simulink model "SIM"  (R2020b)
settings: Solver=ode1  StartTime=0.0  StopTime=inf  FixedStep=0.005  RelTol=1e-3
values from neighbouring files (symbols this model uses):
  previous_input_to_hidden_layer = rand (K,1)* 0.2 - 0.1    [preparation.m]
  TableSIN = [0 0.0549778488291 0.109955562006 0.164933003878 0.219910038795 0.274886531105 0.32986234516 0.384837345313 0.439811395917 0.494784361331 0.549756105914 0.604726494028 ... (5001 elements, 5001x1)]    [TableSIN.mat]
  weights_Qj_model = rand (S,K)* 0.2 - 0.1    [preparation.m]
  weights_W2 = rand ( K+1 , R ) * 0.2 - 0.1    [preparation.m]
  weights_W3 = rand ( R+1 , W ) * 0.2 - 0.1    [preparation.m]
  weights_Wd_model = rand (K,1)* 0.2 - 0.1    [preparation.m]
  weights_Y1_model = rand (K,1)* 0.2 - 0.1    [preparation.m]
  weigths_W1 = rand ( S+1 , K ) * 0.2 - 0.1    [preparation.m]
undefined symbols (not defined in the file or in its folder): D, I, N, P, scaling_a, scaling_b, SkalB, SkalG, strengthening_PID, weights_W1_Model, weights_W2_Model, weights_Xj, WzmocnienieDoWyjscia
libraries: bur_blks x111, pid_lib x3
(part 2 of 2)

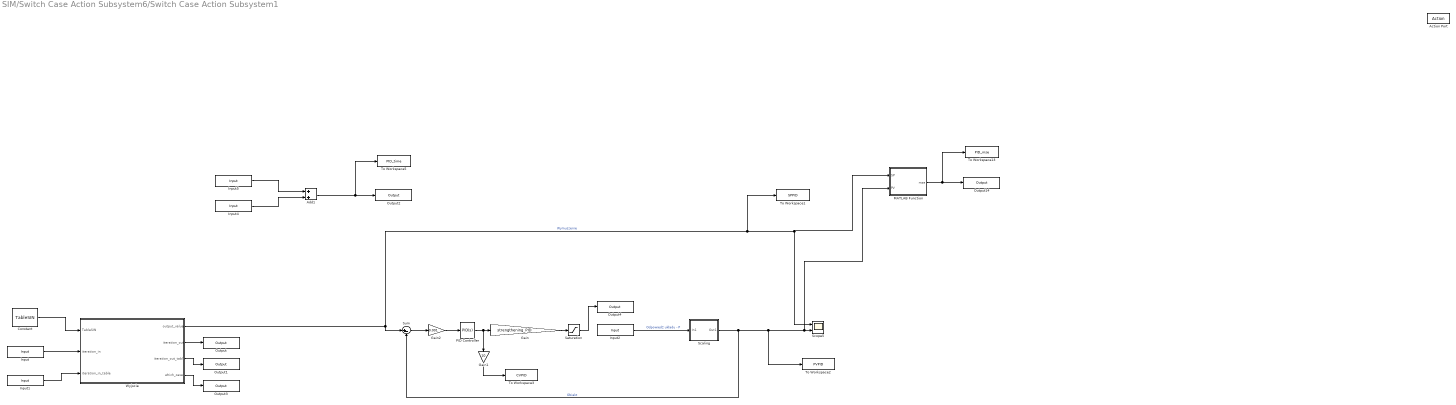
== system SIM/Switch Case Action Subsystem6/Switch Case Action Subsystem1 ==
  Action Port : ActionPort  ActionPortLabel=case [ 2 ]:
  Add1 : Sum
  Constant : Constant  Value=TableSIN
  Gain : Gain  Gain=strengthening_PID
  Gain1 : Gain  Gain=10
  Gain2 : Gain  Gain=0.001
  Input : bur_blks/Input  Tag=LOCAL REAL time_iterator  bur_var_name=time_iterator  bur_scope=LOCAL  bur_data_type=REAL  bur_init_value=-0.001  bur_init_value_bool=FALSE  bur_array_index=0  bur_var_memory=standard  bur_in_parameter=off  bur_AS_string=time_iterator : REAL := -0.001; (**)  bur_array_index_string=0
      settings: AttributesFormatString=%<Tag>  SourceProductName=B&R Automation Studio Toolbox
  Input1 : bur_blks/Input  Tag=LOCAL LREAL table_iterator  bur_var_name=table_iterator  bur_scope=LOCAL  bur_data_type=LREAL  bur_init_value=0  bur_init_value_bool=FALSE  bur_array_index=0  bur_var_memory=standard  bur_in_parameter=off  bur_AS_string=table_iterator : LREAL := 0; (**)  bur_array_index_string=0
      settings: AttributesFormatString=%<Tag>  SourceProductName=B&R Automation Studio Toolbox
  Input2 : bur_blks/Input  Tag=LOCAL LREAL a_input  bur_var_name=a_input  bur_scope=LOCAL  bur_data_type=LREAL  bur_init_value=0  bur_init_value_bool=FALSE  bur_array_index=0  bur_var_memory=standard  bur_in_parameter=off  bur_AS_string=a_input : LREAL := 0; (**)  bur_array_index_string=0
      settings: AttributesFormatString=%<Tag>  SourceProductName=B&R Automation Studio Toolbox
  Input4 : bur_blks/Input  Tag=LOCAL LREAL time  bur_var_name=time  bur_scope=LOCAL  bur_data_type=LREAL  bur_init_value=-0.001  bur_init_value_bool=FALSE  bur_array_index=0  bur_var_memory=standard  bur_in_parameter=off  bur_AS_string=time : LREAL := -0.001; (**)  bur_array_index_string=0
      settings: AttributesFormatString=%<Tag>  SourceProductName=B&R Automation Studio Toolbox
  Input5 : bur_blks/Input  Tag=LOCAL LREAL step  bur_var_name=step  bur_scope=LOCAL  bur_data_type=LREAL  bur_init_value=0  bur_init_value_bool=FALSE  bur_array_index=0  bur_var_memory=standard  bur_in_parameter=off  bur_AS_string=step : LREAL := 0; (**)  bur_array_index_string=0
      settings: AttributesFormatString=%<Tag>  SourceProductName=B&R Automation Studio Toolbox
  MATLAB Function : MATLAB Function  TreatAsAtomicUnit=on
  Output : bur_blks/Output  Tag=LOCAL REAL time_iterator  bur_var_name=time_iterator  bur_scope=LOCAL  bur_data_type=REAL  bur_init_value=0  bur_init_value_bool=FALSE  bur_array_index=0  bur_var_memory=standard  bur_AS_string=time_iterator : REAL := 0; (**)  bur_array_index_string=0
      settings: AttributesFormatString=%<Tag>  SourceProductName=B&R Automation Studio Toolbox
  Output1 : bur_blks/Output  Tag=LOCAL LREAL table_iterator  bur_var_name=table_iterator  bur_scope=LOCAL  bur_data_type=LREAL  bur_init_value=0  bur_init_value_bool=FALSE  bur_array_index=0  bur_var_memory=standard  bur_AS_string=table_iterator : LREAL := 0; (**)  bur_array_index_string=0
      settings: AttributesFormatString=%<Tag>  SourceProductName=B&R Automation Studio Toolbox
  Output14 : bur_blks/Output  Tag=LOCAL LREAL PID_mse  bur_var_name=PID_mse  bur_scope=LOCAL  bur_data_type=LREAL  bur_init_value=0  bur_init_value_bool=FALSE  bur_array_index=0  bur_var_memory=standard  bur_AS_string=PID_mse : LREAL := 0; (**)  bur_array_index_string=0
      settings: AttributesFormatString=%<Tag>  SourceProductName=B&R Automation Studio Toolbox
  Output2 : bur_blks/Output  Tag=LOCAL LREAL time  bur_var_name=time  bur_scope=LOCAL  bur_data_type=LREAL  bur_init_value=0  bur_init_value_bool=FALSE  bur_array_index=0  bur_var_memory=standard  bur_AS_string=time : LREAL := 0; (**)  bur_array_index_string=0
      settings: AttributesFormatString=%<Tag>  SourceProductName=B&R Automation Studio Toolbox
  Output3 : bur_blks/Output  Tag=LOCAL LREAL Case2  bur_var_name=Case2  bur_scope=LOCAL  bur_data_type=LREAL  bur_init_value=0  bur_init_value_bool=FALSE  bur_array_index=0  bur_var_memory=standard  bur_array_index_string=0
      settings: AttributesFormatString=%<Tag>  SourceProductName=B&R Automation Studio Toolbox
  Output4 : bur_blks/Output  Tag=LOCAL LREAL a_output  bur_var_name=a_output  bur_scope=LOCAL  bur_data_type=LREAL  bur_init_value=0  bur_init_value_bool=FALSE  bur_array_index=0  bur_var_memory=standard  bur_AS_string=a_output : LREAL := 0; (**)  bur_array_index_string=0
      settings: AttributesFormatString=%<Tag>  SourceProductName=B&R Automation Studio Toolbox
  PID Controller : pid_lib/PID Controller  Controller=PID  Form=Parallel  TimeDomain=Continuous-time  UseExternalTs=off  SampleTime=-1  IntegratorMethod=Forward Euler  FilterMethod=Forward Euler  ControllerParametersSource=internal  P=P  I=I  D=D  UseFilter=on  N=N  TunerSelectOption=Transfer Function Based (PID Tuner App)  InitialConditionSource=internal  InitialConditionForIntegrator=0  InitialConditionForFilter=0  DifferentiatorICPrevScaledInput=0  ExternalReset=none  TrackingMode=off  Kt=1  LimitOutput=on  SatLimitsSource=internal  UpperSaturationLimit=1  LowerSaturationLimit=-1  LinearizeAsGain=on  AntiWindupMode=clamping  Kb=1  POutMin=[]  POutMax=[]  IOutMin=[]  IOutMax=[]  DOutMin=[]  DOutMax=[]  NOutMin=[]  NOutMax=[]  SumOutMin=[]  SumOutMax=[]  SaturationOutMin=[]  SaturationOutMax=[]  PParamMin=[]  PParamMax=[]  IParamMin=[]  IParamMax=[]  DParamMin=[]  DParamMax=[]  NParamMin=[]  NParamMax=[]  KbParamMin=[]  KbParamMax=[]  KtParamMin=[]  KtParamMax=[]  KbOutMin=[]  KbOutMax=[]  KtOutMin=[]  KtOutMax=[]  IntegratorOutMin=[]  IntegratorOutMax=[]  FilterOutMin=[]  FilterOutMax=[]  SumI1OutMin=[]  SumI1OutMax=[]  SumI2OutMin=[]  SumI2OutMax=[]  SumI3OutMin=[]  SumI3OutMax=[]  SumI4OutMin=[]  SumI4OutMax=[]  SumDOutMin=[]  SumDOutMax=[]  DifferentiatorOutMin=[]  DifferentiatorOutMax=[]  FilterDiffOutCoefMin=[]  FilterDiffOutCoefMax=[]  ReciprocalOutMin=[]  ReciprocalOutMax=[]  SumDenOutMin=[]  SumDenOutMax=[]  SumNumOutMin=[]  SumNumOutMax=[]  DivideOutMin=[]  DivideOutMax=[]  UdiffTsProdOutMin=[]  UdiffTsProdOutMax=[]  NTsProdOutMin=[]  NTsProdOutMax=[]  UintegralTsProdOutMin=[]  UintegralTsProdOutMax=[]  UngainTsProdOutMin=[]  UngainTsProdOutMax=[]  IntegratorContinuousStateAttributes=''  IntegratorStateMustResolveToSignalObject=off  IntegratorRTWStateStorageClass=Auto  FilterContinuousStateAttributes=''  FilterStateMustResolveToSignalObject=off  FilterRTWStateStorageClass=Auto  ParallelPVariant=InternalParameters  IdealPVariant=Disabled  IVariant=InternalParameters  DVariant=InternalParameters  IntegratorVariant=Continuous  SatVariant=Enabled  AWVariant=ContClampingParallel  PCopyVariant=Disabled  TRVariant=Disabled  FdbkBlocksVariant=Forward  IdealPFdbkVariant=Disabled  SatFdbkVariant=Disabled  DerivativeFilterVariant=ContFilter  NVariant=InternalParameters  NCopyVariant=Disabled  FilterICVariant=InternalICsFilter  IntegratorICVariant=InternalICs  ExternalResetVariant=Disabled  TRSumVariant=Passthrough  SumFdbkVariant=Disabled  SumVariant=Sum_PID  TsampFilterVariant=InternalTs  TsampNgainVariant=Passthrough  TsampIntegralVariant=Passthrough  ExternalSaturationOutDataTypeStr=Inherit: Same as second input
  Saturation : Saturate  UpperLimit=32767  LowerLimit=-32767
  Scaling : Subsystem
  Scope5 : Scope  NumInputPorts=2
  Sum : Sum  Inputs=|+-
  To Workspace1 : ToWorkspace  VariableName=SPPID  SampleTime=-1
  To Workspace13 : ToWorkspace  VariableName=PID_mse  SampleTime=-1
  To Workspace2 : ToWorkspace  VariableName=PVPID  SampleTime=-1
  To Workspace3 : ToWorkspace  VariableName=CVPID  SampleTime=-1
  To Workspace5 : ToWorkspace  VariableName=PID_time  SampleTime=-1
  Wyjscie : MATLAB Function  TreatAsAtomicUnit=on
  wires:
  Input4/1 -> Add1/2
  Add1/1 -> To Workspace5/1, Output2/1
  Input5/1 -> Add1/1
  Sum/1 -> Gain2/1
  Wyjscie/1(output_value) -> Sum/1, To Workspace1/1, Scope5/1, MATLAB Function/1(SP)  "Wymuszenie"
  PID Controller/1 -> Gain1/1, Gain/1
  Input/1 -> Wyjscie/2(iteration_in)
  Wyjscie/4(which_case) -> Output3/1
  Wyjscie/3(iteration_out_table) -> Output1/1
  Wyjscie/2(iteration_out) -> Output/1
  Constant/1 -> Wyjscie/1(TableSIN)
  Scaling/1(Out1) -> Sum/2, To Workspace2/1, MATLAB Function/2(PV), Scope5/2  "Obiekt"
  MATLAB Function/1(mse) -> To Workspace13/1, Output14/1
  Input2/1 -> Scaling/1(In1)  "Odpowiedź układu - P"
  Gain/1 -> Saturation/1
  Saturation/1 -> Output4/1
  Gain2/1 -> PID Controller/1
  Gain1/1 -> To Workspace3/1
  Input1/1 -> Wyjscie/3(iteration_in_table)

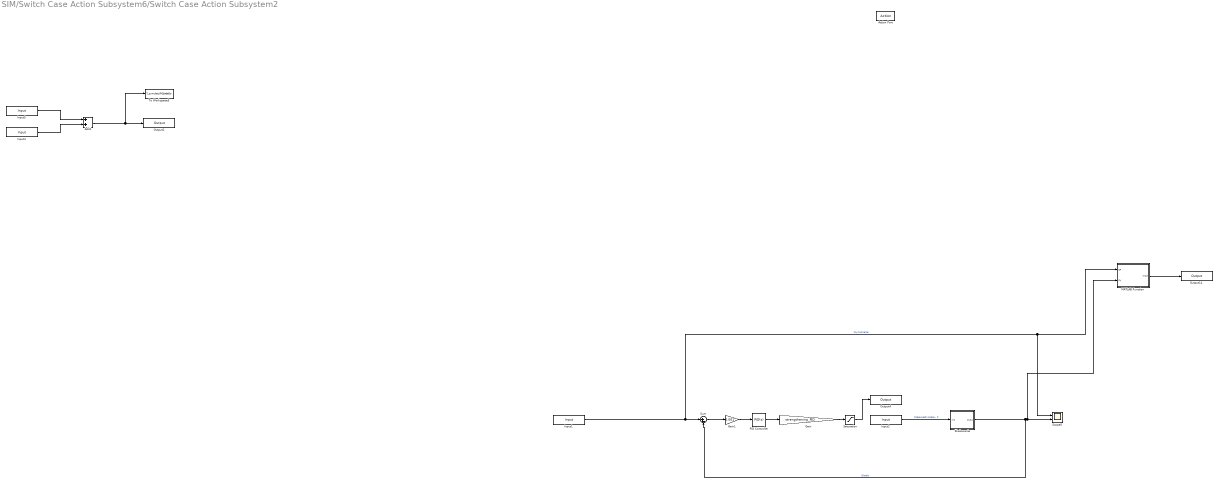
== system SIM/Switch Case Action Subsystem6/Switch Case Action Subsystem2 ==
  Action Port : ActionPort  ActionPortLabel=case [ 3 ]:
  Add1 : Sum
  Gain : Gain  Gain=strengthening_PID
  Gain1 : Gain  Gain=0.001
  Input1 : bur_blks/Input  Tag=LOCAL LREAL PID_reference  bur_var_name=PID_reference  bur_scope=LOCAL  bur_data_type=LREAL  bur_init_value=0  bur_init_value_bool=FALSE  bur_array_index=0  bur_var_memory=standard  bur_in_parameter=off  bur_AS_string=PID_reference : LREAL := 0; (**)  bur_array_index_string=0
      settings: AttributesFormatString=%<Tag>  SourceProductName=B&R Automation Studio Toolbox
  Input2 : bur_blks/Input  Tag=LOCAL LREAL a_input  bur_var_name=a_input  bur_scope=LOCAL  bur_data_type=LREAL  bur_init_value=0  bur_init_value_bool=FALSE  bur_array_index=0  bur_var_memory=standard  bur_in_parameter=off  bur_AS_string=a_input : LREAL := 0; (**)  bur_array_index_string=0
      settings: AttributesFormatString=%<Tag>  SourceProductName=B&R Automation Studio Toolbox
  Input4 : bur_blks/Input  Tag=LOCAL LREAL time  bur_var_name=time  bur_scope=LOCAL  bur_data_type=LREAL  bur_init_value=-0.001  bur_init_value_bool=FALSE  bur_array_index=0  bur_var_memory=standard  bur_in_parameter=off  bur_AS_string=time : LREAL := -0.001; (**)  bur_array_index_string=0
      settings: AttributesFormatString=%<Tag>  SourceProductName=B&R Automation Studio Toolbox
  Input5 : bur_blks/Input  Tag=LOCAL LREAL step  bur_var_name=step  bur_scope=LOCAL  bur_data_type=LREAL  bur_init_value=0  bur_init_value_bool=FALSE  bur_array_index=0  bur_var_memory=standard  bur_in_parameter=off  bur_AS_string=step : LREAL := 0; (**)  bur_array_index_string=0
      settings: AttributesFormatString=%<Tag>  SourceProductName=B&R Automation Studio Toolbox
  MATLAB Function : MATLAB Function  TreatAsAtomicUnit=on
  Output14 : bur_blks/Output  Tag=LOCAL LREAL PID_mse  bur_var_name=PID_mse  bur_scope=LOCAL  bur_data_type=LREAL  bur_init_value=0  bur_init_value_bool=FALSE  bur_array_index=0  bur_var_memory=standard  bur_AS_string=PID_mse : LREAL := 0; (**)  bur_array_index_string=0
      settings: AttributesFormatString=%<Tag>  SourceProductName=B&R Automation Studio Toolbox
  Output2 : bur_blks/Output  Tag=LOCAL LREAL time  bur_var_name=time  bur_scope=LOCAL  bur_data_type=LREAL  bur_init_value=0  bur_init_value_bool=FALSE  bur_array_index=0  bur_var_memory=standard  bur_AS_string=time : LREAL := 0; (**)  bur_array_index_string=0
      settings: AttributesFormatString=%<Tag>  SourceProductName=B&R Automation Studio Toolbox
  Output4 : bur_blks/Output  Tag=LOCAL LREAL a_output  bur_var_name=a_output  bur_scope=LOCAL  bur_data_type=LREAL  bur_init_value=0  bur_init_value_bool=FALSE  bur_array_index=0  bur_var_memory=standard  bur_AS_string=a_output : LREAL := 0; (**)  bur_array_index_string=0
      settings: AttributesFormatString=%<Tag>  SourceProductName=B&R Automation Studio Toolbox
  PID Controller : pid_lib/PID Controller  Controller=PID  Form=Parallel  TimeDomain=Continuous-time  UseExternalTs=off  SampleTime=-1  IntegratorMethod=Forward Euler  FilterMethod=Forward Euler  ControllerParametersSource=internal  P=P  I=I  D=D  UseFilter=on  N=N  TunerSelectOption=Transfer Function Based (PID Tuner App)  InitialConditionSource=internal  InitialConditionForIntegrator=0  InitialConditionForFilter=0  DifferentiatorICPrevScaledInput=0  ExternalReset=none  TrackingMode=off  Kt=1  LimitOutput=on  SatLimitsSource=internal  UpperSaturationLimit=1  LowerSaturationLimit=-1  LinearizeAsGain=on  AntiWindupMode=clamping  Kb=1  POutMin=[]  POutMax=[]  IOutMin=[]  IOutMax=[]  DOutMin=[]  DOutMax=[]  NOutMin=[]  NOutMax=[]  SumOutMin=[]  SumOutMax=[]  SaturationOutMin=[]  SaturationOutMax=[]  PParamMin=[]  PParamMax=[]  IParamMin=[]  IParamMax=[]  DParamMin=[]  DParamMax=[]  NParamMin=[]  NParamMax=[]  KbParamMin=[]  KbParamMax=[]  KtParamMin=[]  KtParamMax=[]  KbOutMin=[]  KbOutMax=[]  KtOutMin=[]  KtOutMax=[]  IntegratorOutMin=[]  IntegratorOutMax=[]  FilterOutMin=[]  FilterOutMax=[]  SumI1OutMin=[]  SumI1OutMax=[]  SumI2OutMin=[]  SumI2OutMax=[]  SumI3OutMin=[]  SumI3OutMax=[]  SumI4OutMin=[]  SumI4OutMax=[]  SumDOutMin=[]  SumDOutMax=[]  DifferentiatorOutMin=[]  DifferentiatorOutMax=[]  FilterDiffOutCoefMin=[]  FilterDiffOutCoefMax=[]  ReciprocalOutMin=[]  ReciprocalOutMax=[]  SumDenOutMin=[]  SumDenOutMax=[]  SumNumOutMin=[]  SumNumOutMax=[]  DivideOutMin=[]  DivideOutMax=[]  UdiffTsProdOutMin=[]  UdiffTsProdOutMax=[]  NTsProdOutMin=[]  NTsProdOutMax=[]  UintegralTsProdOutMin=[]  UintegralTsProdOutMax=[]  UngainTsProdOutMin=[]  UngainTsProdOutMax=[]  IntegratorContinuousStateAttributes=''  IntegratorStateMustResolveToSignalObject=off  IntegratorRTWStateStorageClass=Auto  FilterContinuousStateAttributes=''  FilterStateMustResolveToSignalObject=off  FilterRTWStateStorageClass=Auto  ParallelPVariant=InternalParameters  IdealPVariant=Disabled  IVariant=InternalParameters  DVariant=InternalParameters  IntegratorVariant=Continuous  SatVariant=Enabled  AWVariant=ContClampingParallel  PCopyVariant=Disabled  TRVariant=Disabled  FdbkBlocksVariant=Forward  IdealPFdbkVariant=Disabled  SatFdbkVariant=Disabled  DerivativeFilterVariant=ContFilter  NVariant=InternalParameters  NCopyVariant=Disabled  FilterICVariant=InternalICsFilter  IntegratorICVariant=InternalICs  ExternalResetVariant=Disabled  TRSumVariant=Passthrough  SumFdbkVariant=Disabled  SumVariant=Sum_PID  TsampFilterVariant=InternalTs  TsampNgainVariant=Passthrough  TsampIntegralVariant=Passthrough  ExternalSaturationOutDataTypeStr=Inherit: Same as second input
  Saturation : Saturate  UpperLimit=32767  LowerLimit=-32767
  Scope5 : Scope  NumInputPorts=2
  Skalowanie : Subsystem
  Sum : Sum  Inputs=|+-
  To Workspace5 : ToWorkspace  VariableName=T_symulacjiPIDJadeDo  SampleTime=-1
  wires:
  Input5/1 -> Add1/1
  Add1/1 -> To Workspace5/1, Output2/1
  Input4/1 -> Add1/2
  Sum/1 -> Gain1/1
  MATLAB Function/1(mse) -> Output14/1
  Input1/1 -> MATLAB Function/1(SP), Scope5/1, Sum/1  "Wymuszenie"
  Skalowanie/1(Out1) -> Sum/2, MATLAB Function/2(PV), Scope5/2  "Obiekt"
  Saturation/1 -> Output4/1
  PID Controller/1 -> Gain/1
  Gain/1 -> Saturation/1
  Input2/1 -> Skalowanie/1(In1)  "Odpowiedź układu - P"
  Gain1/1 -> PID Controller/1

== system SIM/Switch Case Action Subsystem6/Switch Case Action Subsystem3 ==
  Action Port : ActionPort  ActionPortLabel=default:
  Constant3 : Constant  Value=-1
  Constant5 : Constant  Value=0
  Constant8 : Constant  Value=-0.001
  Output10 : bur_blks/Output  Tag=LOCAL LREAL time_iterator  bur_var_name=time_iterator  bur_scope=LOCAL  bur_data_type=LREAL  bur_init_value=0  bur_init_value_bool=FALSE  bur_array_index=0  bur_var_memory=standard  bur_AS_string=time_iterator : LREAL := 0; (**)  bur_array_index_string=0
      settings: AttributesFormatString=%<Tag>  SourceProductName=B&R Automation Studio Toolbox
  Output13 : bur_blks/Output  Tag=LOCAL LREAL time  bur_var_name=time  bur_scope=LOCAL  bur_data_type=LREAL  bur_init_value=0  bur_init_value_bool=FALSE  bur_array_index=0  bur_var_memory=standard  bur_AS_string=time : LREAL := 0; (**)  bur_array_index_string=0
      settings: AttributesFormatString=%<Tag>  SourceProductName=B&R Automation Studio Toolbox
  Output9 : bur_blks/Output  Tag=LOCAL LREAL table_sq_iterator  bur_var_name=table_sq_iterator  bur_scope=LOCAL  bur_data_type=LREAL  bur_init_value=0  bur_init_value_bool=FALSE  bur_array_index=0  bur_var_memory=standard  bur_AS_string=table_sq_iterator : LREAL := 0; (**)  bur_array_index_string=0
      settings: AttributesFormatString=%<Tag>  SourceProductName=B&R Automation Studio Toolbox
  wires:
  Constant3/1 -> Output10/1
  Constant5/1 -> Output9/1
  Constant8/1 -> Output13/1

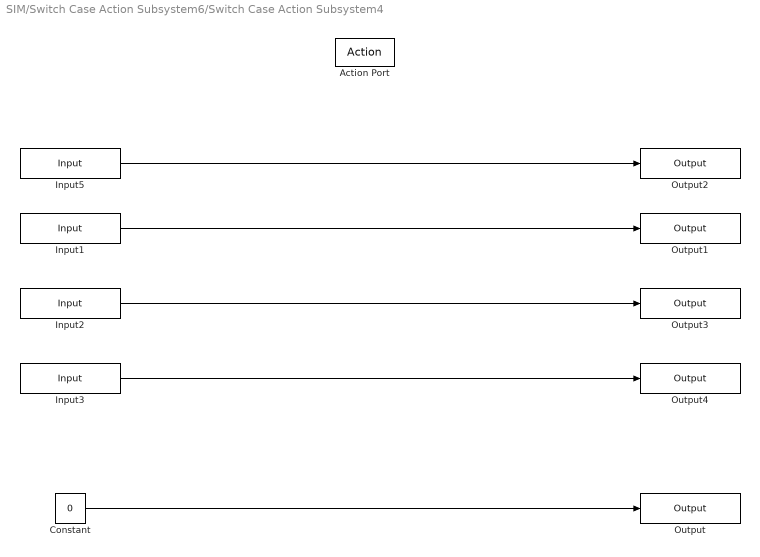
== system SIM/Switch Case Action Subsystem6/Switch Case Action Subsystem4 ==
  Action Port : ActionPort  ActionPortLabel=case [ 1 ]:
  Constant : Constant  Value=0
  Input1 : bur_blks/Input  Tag=LOCAL LREAL new_I  bur_var_name=new_I  bur_scope=LOCAL  bur_data_type=LREAL  bur_init_value=31.35  bur_init_value_bool=FALSE  bur_array_index=0  bur_var_memory=standard  bur_in_parameter=off  bur_AS_string=new_I : LREAL := 31.35; (**)  bur_array_index_string=0
      settings: AttributesFormatString=%<Tag>  SourceProductName=B&R Automation Studio Toolbox
  Input2 : bur_blks/Input  Tag=LOCAL LREAL new_D  bur_var_name=new_D  bur_scope=LOCAL  bur_data_type=LREAL  bur_init_value=0.0076  bur_init_value_bool=FALSE  bur_array_index=0  bur_var_memory=standard  bur_in_parameter=off  bur_AS_string=new_D : LREAL := 0.0076; (**)  bur_array_index_string=0
      settings: AttributesFormatString=%<Tag>  SourceProductName=B&R Automation Studio Toolbox
  Input3 : bur_blks/Input  Tag=LOCAL LREAL new_N  bur_var_name=new_N  bur_scope=LOCAL  bur_data_type=LREAL  bur_init_value=1  bur_init_value_bool=FALSE  bur_array_index=0  bur_var_memory=standard  bur_in_parameter=off  bur_AS_string=new_N : LREAL := 1; (**)  bur_array_index_string=0
      settings: AttributesFormatString=%<Tag>  SourceProductName=B&R Automation Studio Toolbox
  Input5 : bur_blks/Input  Tag=LOCAL LREAL new_P  bur_var_name=new_P  bur_scope=LOCAL  bur_data_type=LREAL  bur_init_value=130  bur_init_value_bool=FALSE  bur_array_index=0  bur_var_memory=standard  bur_in_parameter=off  bur_AS_string=new_P : LREAL := 130; (**)  bur_array_index_string=0
      settings: AttributesFormatString=%<Tag>  SourceProductName=B&R Automation Studio Toolbox
  Output : bur_blks/Output  Tag=LOCAL LREAL Case2  bur_var_name=Case2  bur_scope=LOCAL  bur_data_type=LREAL  bur_init_value=0  bur_init_value_bool=FALSE  bur_array_index=0  bur_var_memory=standard  bur_array_index_string=0
      settings: AttributesFormatString=%<Tag>  SourceProductName=B&R Automation Studio Toolbox
  Output1 : bur_blks/Output  Tag=LOCAL LREAL I  bur_var_name=I  bur_scope=LOCAL  bur_data_type=LREAL  bur_init_value=0  bur_init_value_bool=FALSE  bur_array_index=0  bur_var_memory=standard  bur_array_index_string=0
      settings: AttributesFormatString=%<Tag>  SourceProductName=B&R Automation Studio Toolbox
  Output2 : bur_blks/Output  Tag=LOCAL LREAL P  bur_var_name=P  bur_scope=LOCAL  bur_data_type=LREAL  bur_init_value=0  bur_init_value_bool=FALSE  bur_array_index=0  bur_var_memory=standard  bur_array_index_string=0
      settings: AttributesFormatString=%<Tag>  SourceProductName=B&R Automation Studio Toolbox
  Output3 : bur_blks/Output  Tag=LOCAL LREAL D  bur_var_name=D  bur_scope=LOCAL  bur_data_type=LREAL  bur_init_value=0  bur_init_value_bool=FALSE  bur_array_index=0  bur_var_memory=standard  bur_array_index_string=0
      settings: AttributesFormatString=%<Tag>  SourceProductName=B&R Automation Studio Toolbox
  Output4 : bur_blks/Output  Tag=LOCAL LREAL N  bur_var_name=N  bur_scope=LOCAL  bur_data_type=LREAL  bur_init_value=0  bur_init_value_bool=FALSE  bur_array_index=0  bur_var_memory=standard  bur_array_index_string=0
      settings: AttributesFormatString=%<Tag>  SourceProductName=B&R Automation Studio Toolbox
  wires:
  Constant/1 -> Output/1
  Input5/1 -> Output2/1
  Input1/1 -> Output1/1
  Input2/1 -> Output3/1
  Input3/1 -> Output4/1

== system SIM/Switch Case Action Subsystem4/Switch Case Action Subsystem1/Denormalisation ==
  u : Inport
  Gain1 : Gain  Gain=-1
  Input : bur_blks/Input  Tag=LOCAL LREAL normalisation  bur_var_name=normalisation  bur_scope=LOCAL  bur_data_type=LREAL  bur_init_value=0  bur_init_value_bool=FALSE  bur_array_index=0  bur_var_memory=standard  bur_in_parameter=off  bur_AS_string=normalisation : LREAL := 0; (**)  bur_array_index_string=0
      settings: AttributesFormatString=%<Tag>  SourceProductName=B&R Automation Studio Toolbox
  Input1 : bur_blks/Input  Tag=LOCAL LREAL normalisation  bur_var_name=normalisation  bur_scope=LOCAL  bur_data_type=LREAL  bur_init_value=0  bur_init_value_bool=FALSE  bur_array_index=0  bur_var_memory=standard  bur_in_parameter=off  bur_AS_string=normalisation : LREAL := 0; (**)  bur_array_index_string=0
      settings: AttributesFormatString=%<Tag>  SourceProductName=B&R Automation Studio Toolbox
  MATLAB Function : MATLAB Function  TreatAsAtomicUnit=on
  Xods : Outport
  wires:
  Input1/1 -> Gain1/1
  u/1 -> MATLAB Function/1(Xprze)
  MATLAB Function/1(Xods) -> Xods/1
  Input/1 -> MATLAB Function/2(Xmax)
  Gain1/1 -> MATLAB Function/3(Xmin)

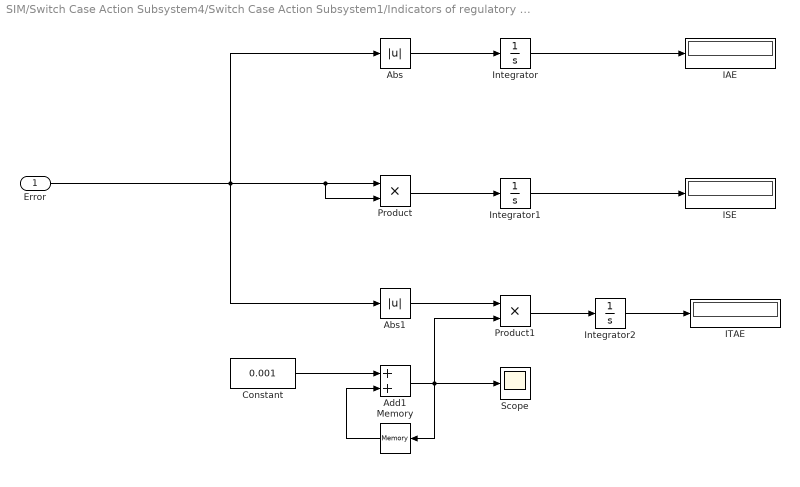
== system SIM/Switch Case Action Subsystem4/Switch Case Action Subsystem1/Indicators of regulatory quality ==
  Error : Inport
  Abs : Abs
  Abs1 : Abs
  Add1 : Sum
  Constant : Constant  Value=0.001
  IAE : Display
  ISE : Display
  ITAE : Display
  Integrator : Integrator
  Integrator1 : Integrator
  Integrator2 : Integrator
  Memory : Memory
  Product : Product
  Product1 : Product
  Scope : Scope
  wires:
  Error/1 -> Abs1/1, Product/2, Product/1, Abs/1
  Abs/1 -> Integrator/1
  Integrator/1 -> IAE/1
  Product/1 -> Integrator1/1
  Integrator1/1 -> ISE/1
  Abs1/1 -> Product1/1
  Constant/1 -> Add1/1
  Add1/1 -> Scope/1, Product1/2, Memory/1
  Product1/1 -> Integrator2/1
  Memory/1 -> Add1/2
  Integrator2/1 -> ITAE/1

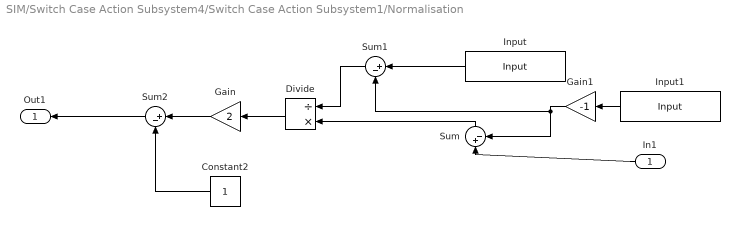
== system SIM/Switch Case Action Subsystem4/Switch Case Action Subsystem1/Normalisation ==
  In1 : Inport
  Constant2 : Constant
  Divide : Product  Inputs=/*
  Gain : Gain  Gain=2
  Gain1 : Gain  Gain=-1
  Input : bur_blks/Input  Tag=LOCAL LREAL normalisation  bur_var_name=normalisation  bur_scope=LOCAL  bur_data_type=LREAL  bur_init_value=0  bur_init_value_bool=FALSE  bur_array_index=0  bur_var_memory=standard  bur_in_parameter=off  bur_AS_string=normalisation : LREAL := 0; (**)  bur_array_index_string=0
      settings: AttributesFormatString=%<Tag>  SourceProductName=B&R Automation Studio Toolbox
  Input1 : bur_blks/Input  Tag=LOCAL LREAL normalisation  bur_var_name=normalisation  bur_scope=LOCAL  bur_data_type=LREAL  bur_init_value=0  bur_init_value_bool=FALSE  bur_array_index=0  bur_var_memory=standard  bur_in_parameter=off  bur_AS_string=normalisation : LREAL := 0; (**)  bur_array_index_string=0
      settings: AttributesFormatString=%<Tag>  SourceProductName=B&R Automation Studio Toolbox
  Sum : Sum  Inputs=|+-
  Sum1 : Sum  Inputs=|+-
  Sum2 : Sum  Inputs=|+-
  Out1 : Outport
  wires:
  In1/1 -> Sum/1
  Divide/1 -> Gain/1
  Sum/1 -> Divide/2
  Sum1/1 -> Divide/1
  Gain/1 -> Sum2/1
  Sum2/1 -> Out1/1
  Constant2/1 -> Sum2/2
  Input/1 -> Sum1/1
  Input1/1 -> Gain1/1
  Gain1/1 -> Sum/2, Sum1/2

== system SIM/Switch Case Action Subsystem4/Switch Case Action Subsystem1/Skalowanie3 ==
  In1 : Inport
  Add : Sum
  Constant : Constant  Value=SkalB
  Gain : Gain  Gain=SkalG
  Out1 : Outport
  wires:
  In1/1 -> Gain/1
  Gain/1 -> Add/2
  Add/1 -> Out1/1
  Constant/1 -> Add/1

== system SIM/Switch Case Action Subsystem6/Switch Case Action Subsystem1/Scaling ==
  In1 : Inport
  Add : Sum
  Constant : Constant  Value=scaling_b
  Gain : Gain  Gain=scaling_a
  Out1 : Outport
  wires:
  In1/1 -> Gain/1
  Gain/1 -> Add/2
  Add/1 -> Out1/1
  Constant/1 -> Add/1

== system SIM/Switch Case Action Subsystem6/Switch Case Action Subsystem2/Skalowanie ==
  In1 : Inport
  Add : Sum
  Constant : Constant  Value=scaling_b
  Gain : Gain  Gain=scaling_a
  Out1 : Outport
  wires:
  In1/1 -> Gain/1
  Gain/1 -> Add/2
  Add/1 -> Out1/1
  Constant/1 -> Add/1

== matlab function SIM/Switch Case Action Subsystem/MATLAB Function ==
  data: u input; max_output output; max_actual_output input; min_actual_output input; min_output output
function [max_output,min_output] = fcn(u,max_actual_output,min_actual_output)

max_output = max_actual_output;
min_output = min_actual_output;

if max_actual_output < u
   
    max_output = u;
    
end

if min_actual_output > u
   
    min_output = u;

end

    
end

== matlab function SIM/Switch Case Action Subsystem3/MATLAB Function ==
  data: scaling_a output; max_output input; min_output input; scaling_b output; which_case output
function [scaling_a,scaling_b,which_case] = fcn(max_output,min_output)

MAX = 67.75;
MIN = -67.75;

scaling_a = (MAX-MIN)/(max_output - min_output);
scaling_b = MAX - scaling_a*max_output;

which_case = 0;

end

== matlab function SIM/Switch Case Action Subsystem2/MATLAB Function1 ==
  data: T_symulacji input; Czy_koniec output
function Czy_koniec = fcn(T_symulacji)

Czy_koniec = 0;

if T_symulacji > 3
    
    Czy_koniec = 1;
end

== matlab function SIM/Switch Case Action Subsystem4/Switch Case Action Subsystem1/DRNN ==
  data: E input; reference_signal input; y output; weights_W1 input; weights_W2 input; weights_Wd_model input; weights_Xj_model input; previous_input_to_hidden_layer input; weights_Qj_model input; weights_W1_after output; weights_W2_after output; weights_Wd_after output; MSEOUT output; Xj_after output; Pj_after output; Qj_after output; previous_output_of_object_d1 input; previous_output_of_object_d2 input; iteration_before input; iteration_after output; output_of_hidden_layer output
function [y,weights_W1_after,weights_W2_after, weights_Wd_after,MSEOUT,Xj_after,Pj_after,Qj_after,iteration_after,output_of_hidden_layer] = ...
    fcn(E,reference_signal,weights_W1,weights_W2,weights_Wd_model,weights_Xj_model,previous_input_to_hidden_layer,weights_Qj_model,...
    previous_output_of_object_d1,previous_output_of_object_d2,iteration_before)

function [ W1po, W2po, Wdpo, MSE ] = ucz2 ( weights_W1_before , weights_W2_before , weights_Wd_before , input_to_network, previous_input_to_hidden_layer, Qjd , Xjd)
W1 = weights_W1_before ;
W2 = weights_W2_before ;
Wd = weights_Wd_before;
Xj = Xjd;

X = input_to_network; % wejścia sieci
[ Y1 , Y2, Xjpo] = dzialaj2 ( W1 , W2 , Wd , X , Xj) ;
X1 = [ X ] ; % wejścia warstwy 1
X2 = [ Y1 ] ; % wejścia warstwy 2
D2 = E; % oblicz błędy dla warstwy 2
E2 = D2; % błąd„wewnętrzny” warstwy 2
MSE = 0.5*D2'*D2;

coefficient = 1.5;
countofneurons = 15;

DerivativeUcAfterW2 = X2;
dW2 = DerivativeUcAfterW2;
W2 = W2 + (coefficient/(countofneurons))*dW2*E2';
wspUcz2warstwy = coefficient/(countofneurons);

W2max = max(abs(W2));
Imax = max(abs(X));

DerivativeUcAfterWd = (1 - Y1.*Y1);
%dWd = DerivativeUcAfterWd.*(Xjd + Wd.*Pjd);
dWd = (Xjd + previous_input_to_hidden_layer.*Wd).*(DerivativeUcAfterWd.*W2);
Pj_after = dWd;
Wd = Wd + (coefficient/(countofneurons*W2max*W2max))*dWd*E2;
wspUczPetli = coefficient/(countofneurons*W2max*W2max);
Wd(Wd>1)=1;
Wd(Wd<-1)=-1;

DerivativeUcAfterW1 = (1 - Y1.*Y1);
dW1 = (X1 + Qjd*Wd)*(DerivativeUcAfterW1.*W2)';
Qj_after = dW1;
W1 = W1 + (coefficient/(countofneurons*W2max*W2max*Imax*Imax))*dW1*E2;
wspUcz1warstwy = coefficient/(countofneurons*W2max*W2max*Imax*Imax);

W1po = W1 ;
W2po = W2 ;
Wdpo = Wd;

end

function [ Y1 , Y2, Xjpo ] = dzialaj2 ( W1 , W2, Wd , X , Xjd)
X1 = [ X ] ;
U1 = W1' * X1 + Wd'*Xjd;
Y1 = tanh(U1);
Xjpo = Y1;
X2 = [ Y1 ] ;
U2 = W2' * X2 ;
Y2 = U2;
end

P = [reference_signal;previous_output_of_object_d1;previous_output_of_object_d2];

[ W1po , W2po, Wdpo, MSE ] = ucz2( weights_W1 , weights_W2, weights_Wd_model , P, previous_input_to_hidden_layer, weights_Qj_model ,weights_Xj_model);

[ Y1 , Y2, Xjpo ] = dzialaj2( W1po , W2po, Wdpo , P , weights_Xj_model) ;

Xj_after = Xjpo;
weights_W1_after = W1po;
weights_W2_after = W2po;
weights_Wd_after = Wdpo;
MSEOUT = MSE;

iteration_after = iteration_before + 1;

y = Y2;
output_of_hidden_layer = Y1;

end

== matlab function SIM/Switch Case Action Subsystem4/Switch Case Action Subsystem1/Denormalisation/MATLAB Function ==
  data: Xprze input; Xods output; Xmax input; Xmin input
function Xods = fcn(Xprze, Xmax, Xmin)

Xods = (Xprze+1)/2*(Xmax-Xmin) + Xmin;

== matlab function SIM/Switch Case Action Subsystem4/Switch Case Action Subsystem1/NARX - Lypunov learning rate old bias HDLNNC - 3 layers7 ==
  data: E input; ud1 input; ud2 input; ud3 input; u output; old_weights_W1_HDL input; old_weights_W2_HDL input; old_weights_W3_HDL input; new_weights_W1_HDL output; new_weights_W2_HDL output; new_weights_W3_HDL output; MSEOUT output; iteration_before input; iteration_after_calculation output; weights_of_DRNN_W1 input; output_of_model input; weights_of_DRNN_W2 input; previous_output input; total_iteration input
function [u,new_weights_W1_HDL,new_weights_W2_HDL,new_weights_W3_HDL,MSEOUT,iteration_after_calculation] = ...
    fcn(E,ud1,ud2,ud3,old_weights_W1_HDL,old_weights_W2_HDL,old_weights_W3_HDL,...
    iteration_before,weights_of_DRNN_W1,output_of_model,weights_of_DRNN_W2,previous_output,total_iteration)

function [output_of_frist_layer,new_weights_W1_HDL] = f_teach_HDL_first_layer(old_weights_W1_HDL,P)
    number_of_neurons = size(old_weights_W1_HDL,2);
    new_weights_W1_HDL = old_weights_W1_HDL;
    min_distance = 1000;
    min_index = 1;
    X = [-1;P];
    for iteration = 1:number_of_neurons
        actual_neuron = new_weights_W1_HDL(:,iteration);
        actual_difference = abs(X-actual_neuron);
        sum_of_actual_difference = sum(actual_difference);
        if sum_of_actual_difference < min_distance
            min_distance = sum_of_actual_difference;
            min_index = iteration;
        end
    end
    
    l_0 = 0.00000005;
    %l_0 = 0.00005;
        
    l = l_0*2.718^(-iteration_before/total_iteration);

    ki_0 = 0.000007;
    ki_f = 0.000005;
    which_iteration = iteration_before/total_iteration;
    sigma = ki_0*(-((ki_f/ki_0).^(which_iteration)));
    
    for iteration = 1:number_of_neurons 
        ro = l*2.718.^(-((power(new_weights_W1_HDL(:,min_index)-new_weights_W1_HDL(:,iteration),2)))/(2*sigma*sigma));
        pom_ro = find(ro>1);
        ro(pom_ro) = 1;
        pom_ro = find(ro<0);
        ro(pom_ro) = 0;
        update = ro.*(X - new_weights_W1_HDL(:,iteration));
        new_weights_W1_HDL(:,iteration) = old_weights_W1_HDL(:,iteration) + update;
    end
    
    U1 = new_weights_W1_HDL' * X;
    output_of_frist_layer = tanh(U1);
end

function [output_of_second_layer,new_weights_W2_HDL] = f_teach_HDL_second_layer(old_weights_W2_HDL,input)
  number_of_neurons = size(old_weights_W2_HDL,2);
  new_weights_W2_HDL = old_weights_W2_HDL;
  min_distance = 1000;
  min_index = 1;
  X = [-1;input];
  
  for iteration = 1:number_of_neurons
        actual_neuron = new_weights_W2_HDL(:,iteration);
        actual_difference = abs(X-actual_neuron);
        sum_of_actual_difference = sum(actual_difference);
        if sum_of_actual_difference < min_distance
            min_distance = sum_of_actual_difference;
            min_index = iteration;
        end
  end
  
  l_0 = 0.00000005;

  l = l_0*2.718^(-iteration_before/total_iteration);

  ki_0 = 0.000007;
  ki_f = 0.000005;
  which_iteration = iteration_before/total_iteration;
  sigma = ki_0*(-power((ki_f/ki_0),(which_iteration)));
  
  
for iteration = 1:number_of_neurons
    ro = l*exp(-(power(new_weights_W2_HDL(:,min_index)-new_weights_W2_HDL(:,iteration),2))/(2*sigma*sigma));
    pom_ro = find(ro>1);
    ro(pom_ro) = 1;
    pom_ro = find(ro<0);
    ro(pom_ro) = 0;
    update = ro.*(X - new_weights_W2_HDL(:,iteration));
    new_weights_W2_HDL(:,iteration) = old_weights_W2_HDL(:,iteration) + update;
end
  
  U2 = new_weights_W2_HDL' * X;
  output_of_second_layer = tanh(U2);
end

function [new_weights_W3_HDL] = f_teach_HDL_thrid_layer(old_weights_W3_HDL,output_of_second_layer)
    alpha = 0.0001;
    eta = 0.000001;
    new_weights_W3_HDL = old_weights_W3_HDL + alpha*previous_output*[-1;output_of_second_layer] - eta*previous_output*old_weights_W3_HDL;
end

function [ new_weights_W3 , new_weights_W2, new_weights_W1, MSE] = f_teach_MLP (W1 , W2, W3, P)
number_of_neurons_second_layer = size(W2,1) ;
number_of_neurons_third_layer = size(W3,1) ;

X = P; % entry into the network
[ Y1 , Y2, Y3 ] = f_calculate_the_output_of_NN ( W1 , W2, W3 , X ) ;
X1 = [ -1 ; X ] ; % input to layer one
X2 = [ -1 ; Y1 ] ; % input to layer two
X3 = [ -1 ; Y2]; % input to layer third
D3 = satlin_moj(E); % error of control
MSE = 0.5*D3'*D3; %value of MSE

derivative_yp_of_u =abs((weights_of_DRNN_W2.*(1-output_of_model.*output_of_model))'*(weights_of_DRNN_W1(1,:))');

derivative_u_of_w3 = X3;

beta = 0.7;
delta = 1;

sigma = 0.0009;

eta_layer_3 = sigma./(delta.*(1+beta/delta*(E3.*derivative_u_of_w3.*derivative_yp_of_u).^2)); % learning coefficient layer 3

dW3 = eta_layer_3.*E3.*derivative_yp_of_u.*derivative_u_of_w3; % derivative of layer 3

W3 = W3 + dW3; % update of layer 3 weights

%Second Layer

derivative_u_of_w2 = X2*(W3(2:number_of_neurons_third_layer,:).*(1-Y2.*Y2))';

eta_layer_2 = sigma./(delta.*(1+beta/delta*(E3.*derivative_u_of_w2.*derivative_yp_of_u).^2)); % learning coefficient layer 2

dW2 = eta_layer_2.*derivative_u_of_w2.*derivative_yp_of_u.*E3; % derivative of layer 2

W2 = W2 + dW2; % update of layer 2 weights

%First Layer

derivative_u_of_w1 = X1*(((W3(2:number_of_neurons_third_layer,:).*(1-Y2.*Y2))'*W2(2:number_of_neurons_second_layer,:)').*(1-Y1.*Y1)');

eta_layer_1 = sigma./(delta.*(1+beta/delta*(E3.*derivative_u_of_w1.*derivative_yp_of_u).^2)); % learning coefficient layer 1

dW1 = eta_layer_1.*derivative_u_of_w1.*derivative_yp_of_u.*E3; % derivative of layer 1

W1 = W1 + dW1; % update of layer 1 weights

new_weights_W3 = W1 ; %new weights
new_weights_W2 = W2 ; %new weights
new_weights_W1 = W3 ; %new weights

end

function [ Y1 , Y2 , Y3 ] = f_calculate_the_output_of_NN ( W1 , W2, W3, P)
X1 = [ -1; P ] ;
U1 = W1' * X1 ;
Y1 = tanh(U1);

X2 = [ -1; Y1 ] ;
U2 = W2' * X2 ;
Y2 = tanh(U2);

X3 = [ -1; Y2 ] ;
U3 = W3' * X3 ;
Y3 = satlin_moj(U3);
Y3 = U3;
end

function [Y] = satlin_moj(X)
    
    if X<1 & X>-1
        Y=X;
    elseif X > 1
        Y=1;
    elseif X<-1
        Y=-1;
    else
        Y=0;
    end
end

P = [ud1;ud2;ud3]; %input

[OutputOfFirstLayer,new_weights_W1_HDL] = f_teach_HDL_first_layer(old_weights_W1_HDL,P);

[output_of_second_layer,new_weights_W2_HDL] = f_teach_HDL_second_layer(old_weights_W2_HDL,OutputOfFirstLayer);

[new_weights_W3_HDL] = f_teach_HDL_thrid_layer(old_weights_W3_HDL,output_of_second_layer);

[ new_weights_W3 , W2po, W3po, MSE ] = f_teach_MLP( new_weights_W1_HDL , new_weights_W2_HDL, new_weights_W3_HDL , P);

[ Y1 , Y2 , Y3 ] = f_calculate_the_output_of_NN( new_weights_W1_HDL , new_weights_W2_HDL, new_weights_W3_HDL , P) ;

u = satlin_moj(Y3);

new_weights_W1_HDL = new_weights_W3; %new weights
new_weights_W2_HDL = W2po; %new weights
new_weights_W3_HDL = W3po; %new weights

MSEOUT = MSE;

iteration_after_calculation = iteration_before + 1;

end

== matlab function SIM/Switch Case Action Subsystem4/Switch Case Action Subsystem1/Wyjscie5 ==
  data: TableSIN input; output_value output; iteration_in input; iteration_out output; iteration_in_table input; iteration_out_table output; which_case output
function [output_value,iteration_out, iteration_out_table, which_case] = ...
    oblicz_wyjscie(TableSIN, iteration_in, iteration_in_table)

output_value = 0;
which_case = 2;

iteration_out_table = iteration_in_table;

if iteration_in<49999 
    output_value = TableSIN(iteration_in_table,1);

    iteration_out_table = iteration_in_table + 1;

    if iteration_out_table > 4999
        iteration_out_table = 1;
    end

elseif iteration_in>=49999 
    which_case = 0;
end

iteration_out = iteration_in + 1;


end

== matlab function SIM/Switch Case Action Subsystem6/Switch Case Action Subsystem1/Wyjscie ==
  data: TableSIN input; output_value output; iteration_in input; iteration_in_table input; iteration_out output; iteration_out_table output; which_case output
function [output_value,iteration_out, iteration_out_table, which_case] = ...
    oblicz_wyjscie(TableSIN, iteration_in, iteration_in_table)

output_value = 0;
which_case = 2;

iteration_out_table = iteration_in_table;

if iteration_in<49999 
    output_value = TableSIN(iteration_in_table,1);

    iteration_out_table = iteration_in_table + 1;

    if iteration_out_table > 4999
        iteration_out_table = 1;
    end

elseif iteration_in>=49999 
    which_case = 0;
end

iteration_out = iteration_in + 1;


end

== matlab function SIM/Switch Case Action Subsystem6/Switch Case Action Subsystem1/MATLAB Function ==
  data: SP input; mse output; PV input
function mse = fcn(SP,PV)

mse = (SP-PV)*(SP-PV)/2;

end

== matlab function SIM/Switch Case Action Subsystem6/Switch Case Action Subsystem2/MATLAB Function ==
  data: SP input; mse output; PV input
function mse = fcn(SP,PV)

mse = (SP-PV)*(SP-PV)/2;

end

== matlab function SIM/Switch Case Action Subsystem14/MATLAB Function ==
  data: time input; u output; which_case output
function [u,which_case] = fcn(time)

u = 1;
which_case = 7;

if time<0.5
    u = 0;
elseif time<0.8
    u = 1;
elseif time<2
    u = 0;
else
    u = 0;
    which_case = 0;
end

end

== matlab function SIM/Switch Case Action Subsystem/MATLAB Function1 ==
  data: y output; which_case output; time input
function [y,which_case] = fcn(time)

which_case = 1;

if time < 5
    
    u = 1;
    
elseif time >= 5 && time < 10
    
    u = -1;
else
    u = 0;
    which_case = 2;
end

y = u;
